simulink model "Motor_model"  (R2018a)
settings: Solver=VariableStepAuto  StartTime=0.0  StopTime=50
values from neighbouring files (symbols this model uses):
  a = Rr/Lr    (= 342.760962802)    [IM_model.m]
  b = Msr/(sigma*Ls*Lr)    (= -1.03784964259)    [IM_model.m]
  c = f/J    (= 0.00909090909091)    [IM_model.m]
  gamma = ((Lr^2)*Rs+Msr^2)/(sigma*Ls*(Lr^2))    (= -33.4582958771)    [IM_model.m]
  J = 0.011    [IM_model.m]    (also in transfer_function.m)
  m = p*Msr/(J*Lr)    (= 2899.38130148)    [IM_model.m]
  m1 = 1/(sigma*Ls)    (= -0.0325414140802)    [IM_model.m]
  Msr = 0.9644789    [IM_model.m]    (also in transfer_function.m)
  p = 1    [IM_model.m]    (also in transfer_function.m)
  ws = 2*pi*fs    (= 314.159265359)    [IM_model.m]
libraries: powerlib_meascontrol x3, powerlib x1
settings Model: Creator=ali  LastModifiedBy=ali

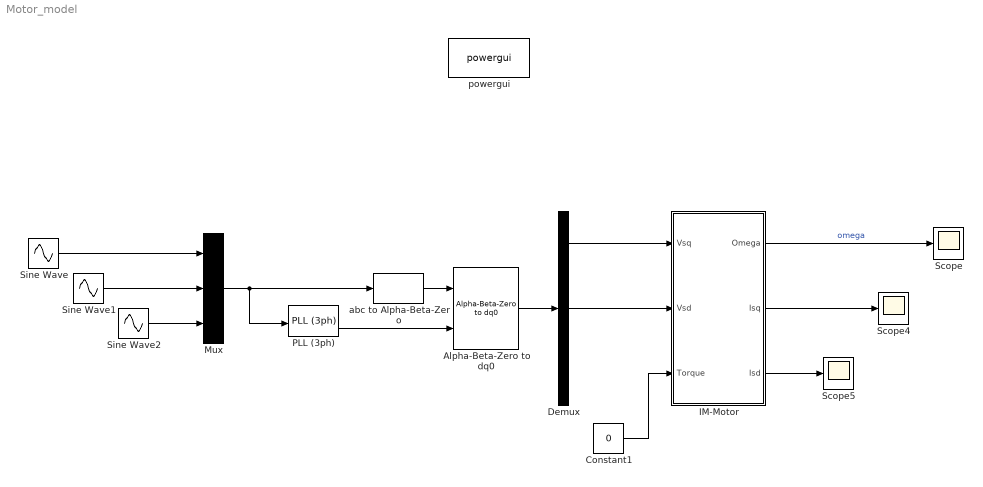
== system Motor_model ==
  Alpha-Beta-Zero to dq0 : powerlib_meascontrol/Transformations/Alpha-Beta-Zero to dq0  Alignment=90 degrees behind phase A axis
      settings: SourceProductName=Simscape Power Systems
  Constant1 : Constant  Value=0
  Demux : Demux  Outputs=3
  IM-Motor : Subsystem
  Mux : Mux  Inputs=3
  PLL (3ph) : powerlib_meascontrol/PLL/PLL (3ph)  Fmin=45  Par_Init=[0, 50]  ParK=[180, 3200, 1]  TcD=1e-4  MaxRateChangeFreq=12  FilterCutOffFreq=25  Ts=0  AGC=on
  Scope : Scope
  Scope4 : Scope
  Scope5 : Scope
  Sine Wave : Sin  Amplitude=220*sqrt(2)  Frequency=2*pi*50  SampleTime=0
  Sine Wave1 : Sin  Amplitude=220*sqrt(2)  Frequency=2*pi*50  Phase=(-120)*(2*pi/360)  SampleTime=0
  Sine Wave2 : Sin  Amplitude=220*sqrt(2)  Frequency=2*pi*50  Phase=(-240)*(2*pi/360)  SampleTime=0
  abc to Alpha-Beta-Zero : powerlib_meascontrol/Transformations/abc to Alpha-Beta-Zero
      settings: SourceProductName=Simscape Power Systems
  powergui : powerlib/powergui  Priority=1  SimulationMode=Continuous  SampleTime=50e-6  frequency=60  Iterations=50  frequencyindice=60  Pbase=100e6  ErrMax=1e-4  UnitsV=kV  UnitsW=MW  buscounter=0  FunctionMessages=off  echomessages=off  EnableUseOfTLC=off  CurrentSourceSwitches=off  DisableSnubberDevices=off  DisableRonSwitches=off  DisableVfSwitches=off  DisplayEquations=off  SolverType=Tustin/Backward Euler (TBE)  Interpol=off  ExternalGateDelay=off  methode=off  Ts=100  x0status=blocks  SPID=on  SwTol=0  HookPort=off  RestoreLinks=warning  ResistiveCurrentMeasurement=off  Frange=[0:2:500]  Ylog=off  Xlog=on  ShowGrid=off  save=off  variable=ZData  structure=0  ZoomFFT=off  StartTime=0.0  cycles=1  DisplayStyle=1  fundamental=60  FreqAxis=off  MaxFrequency=1000  frequencyindicesteady=1  RmsSteady=1  display=off
  wires:
  IM-Motor/1(Omega) -> Scope/1  "omega"
  Sine Wave/1 -> Mux/1
  Sine Wave1/1 -> Mux/2
  Sine Wave2/1 -> Mux/3
  Constant1/1 -> IM-Motor/3(Torque)
  Mux/1 -> abc to Alpha-Beta-Zero/1, PLL (3ph)/1
  abc to Alpha-Beta-Zero/1 -> Alpha-Beta-Zero to dq0/1
  PLL (3ph)/2 -> Alpha-Beta-Zero to dq0/2
  IM-Motor/2(Isq) -> Scope4/1
  IM-Motor/3(Isd) -> Scope5/1
  Alpha-Beta-Zero to dq0/1 -> Demux/1
  Demux/1 -> IM-Motor/1(Vsq)
  Demux/2 -> IM-Motor/2(Vsd)

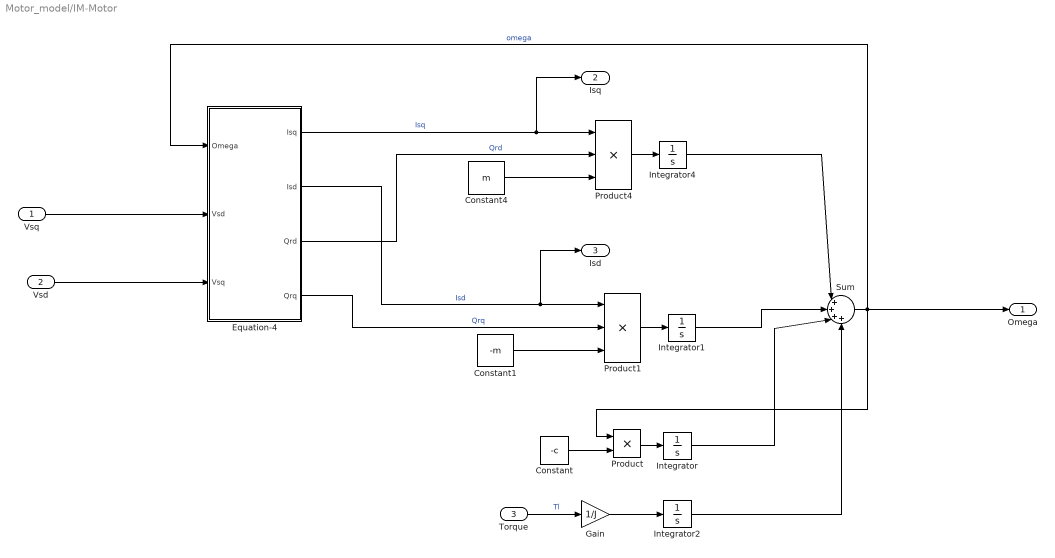
== system Motor_model/IM-Motor ==
  Vsq : Inport
  Vsd : Inport  Port=2
  Torque : Inport  Port=3
  Constant : Constant  Value=-c
  Constant1 : Constant  Value=-m
  Constant4 : Constant  Value=m
  Equation-4 : Subsystem
  Gain : Gain  Gain=1/J
  Integrator{,1..2,4} (4 alike) : Integrator
  Product : Product
  Product1 : Product  Inputs=3
  Product4 : Product  Inputs=3
  Sum : Sum  Inputs=|++++
  Omega : Outport
  Isq : Outport  Port=2
  Isd : Outport  Port=3
  wires:
  Equation-4/1(Isq) -> Isq/1, Product4/1  "Isq"
  Product/1 -> Integrator/1
  Sum/1 -> Omega/1, Equation-4/1(Omega), Product/1  "omega"
  Integrator/1 -> Sum/3
  Integrator4/1 -> Sum/1
  Constant/1 -> Product/2
  Integrator1/1 -> Sum/2
  Equation-4/3(Qrd) -> Product4/2  "Qrd"
  Vsq/1 -> Equation-4/2(Vsd)
  Equation-4/2(Isd) -> Isd/1, Product1/1  "Isd"
  Vsd/1 -> Equation-4/3(Vsq)
  Constant4/1 -> Product4/3
  Equation-4/4(Qrq) -> Product1/2  "Qrq"
  Product4/1 -> Integrator4/1
  Constant1/1 -> Product1/3
  Product1/1 -> Integrator1/1
  Integrator2/1 -> Sum/4
  Gain/1 -> Integrator2/1
  Torque/1 -> Gain/1  "Tl"

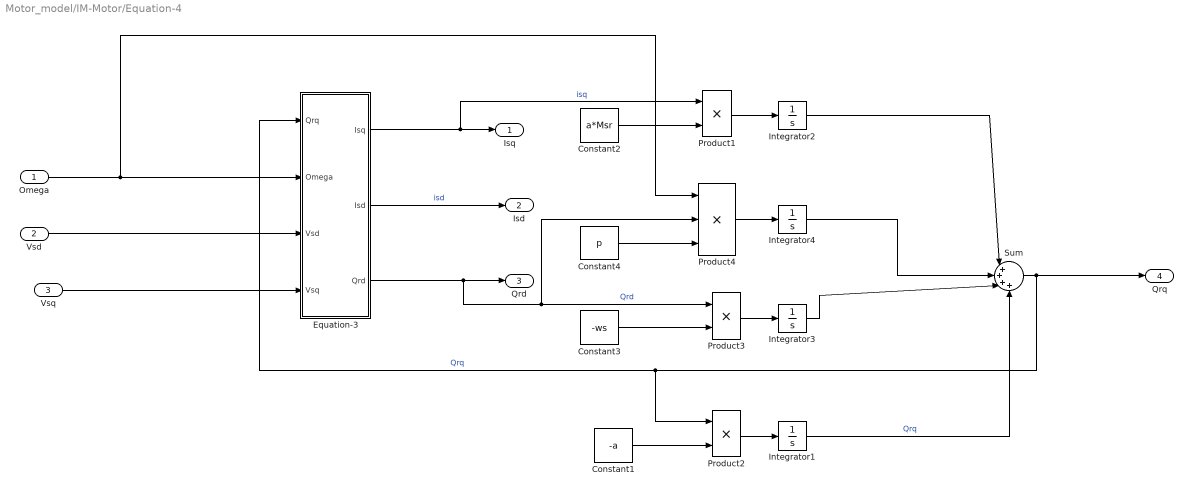
== system Motor_model/IM-Motor/Equation-4 ==
  Omega : Inport
  Vsd : Inport  Port=2
  Vsq : Inport  Port=3
  Constant1 : Constant  Value=-a
  Constant2 : Constant  Value=a*Msr
  Constant3 : Constant  Value=-ws
  Constant4 : Constant  Value=p
  Equation-3 : Subsystem
  Integrator{1..4} (4 alike) : Integrator
  Product1 : Product
  Product2 : Product
  Product3 : Product
  Product4 : Product  Inputs=3
  Sum : Sum  Inputs=|++++
  Isq : Outport
  Isd : Outport  Port=2
  Qrd : Outport  Port=3
  Qrq : Outport  Port=4
  wires:
  Product3/1 -> Integrator3/1
  Equation-3/3(Qrd) -> Qrd/1, Product4/2, Product3/1  "Qrd"
  Product2/1 -> Integrator1/1
  Constant2/1 -> Product1/2
  Sum/1 -> Qrq/1, Product2/1, Equation-3/1(Qrq)  "Qrq"
  Integrator2/1 -> Sum/1
  Omega/1 -> Product4/1, Equation-3/2(Omega)
  Integrator4/1 -> Sum/2
  Constant3/1 -> Product3/2
  Integrator3/1 -> Sum/3
  Product1/1 -> Integrator2/1
  Integrator1/1 -> Sum/4  "Qrq"
  Constant4/1 -> Product4/3
  Vsd/1 -> Equation-3/3(Vsd)
  Vsq/1 -> Equation-3/4(Vsq)
  Equation-3/2(Isd) -> Isd/1  "isd"
  Equation-3/1(Isq) -> Isq/1, Product1/1  "isq"
  Product4/1 -> Integrator4/1
  Constant1/1 -> Product2/2

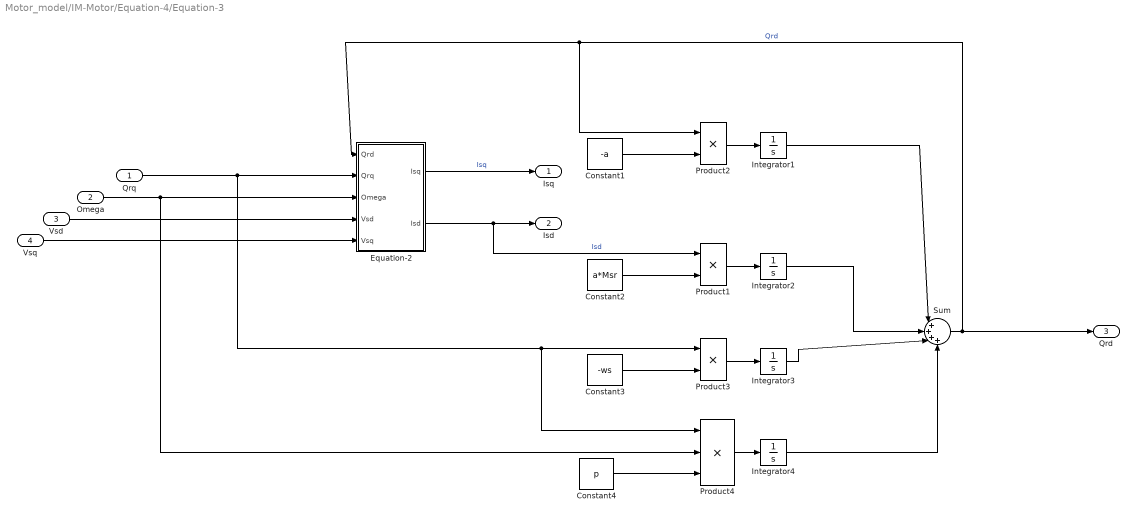
== system Motor_model/IM-Motor/Equation-4/Equation-3 ==
  Qrq : Inport
  Omega : Inport  Port=2
  Vsd : Inport  Port=3
  Vsq : Inport  Port=4
  Constant1 : Constant  Value=-a
  Constant2 : Constant  Value=a*Msr
  Constant3 : Constant  Value=-ws
  Constant4 : Constant  Value=p
  Equation-2 : Subsystem
  Integrator{1..4} (4 alike) : Integrator
  Product1 : Product
  Product2 : Product
  Product3 : Product
  Product4 : Product  Inputs=3
  Sum : Sum  Inputs=|++++
  Isq : Outport
  Isd : Outport  Port=2
  Qrd : Outport  Port=3
  wires:
  Vsd/1 -> Equation-2/4(Vsd)
  Product4/1 -> Integrator4/1
  Qrq/1 -> Equation-2/2(Qrq), Product4/1, Product3/1
  Sum/1 -> Qrd/1, Equation-2/1(Qrd), Product2/1  "Qrd"
  Integrator2/1 -> Sum/2
  Integrator1/1 -> Sum/1
  Omega/1 -> Product4/2, Equation-2/3(Omega)
  Integrator3/1 -> Sum/3
  Equation-2/2(Isd) -> Isd/1, Product1/1  "Isd"
  Integrator4/1 -> Sum/4
  Constant2/1 -> Product1/2
  Constant4/1 -> Product4/3
  Product3/1 -> Integrator3/1
  Constant3/1 -> Product3/2
  Constant1/1 -> Product2/2
  Equation-2/1(Isq) -> Isq/1  "Isq"
  Product2/1 -> Integrator1/1
  Product1/1 -> Integrator2/1
  Vsq/1 -> Equation-2/5(Vsq)

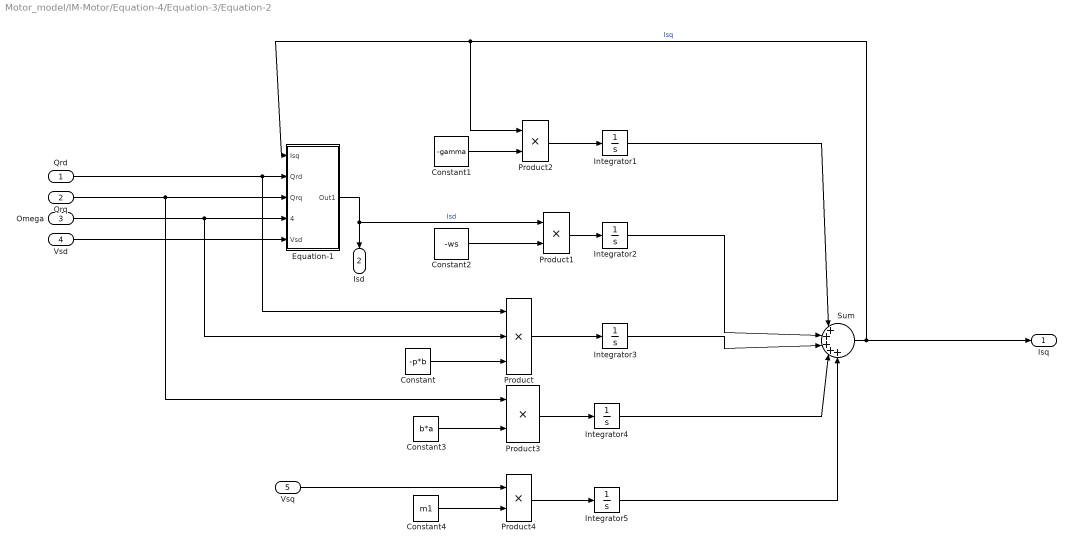
== system Motor_model/IM-Motor/Equation-4/Equation-3/Equation-2 ==
  Qrd : Inport
  Qrq : Inport  Port=2
  Omega : Inport  Port=3
  Vsd : Inport  Port=4
  Vsq : Inport  Port=5
  Constant : Constant  Value=-p*b
  Constant1 : Constant  Value=-gamma
  Constant2 : Constant  Value=-ws
  Constant3 : Constant  Value=b*a
  Constant4 : Constant  Value=m1
  Equation-1 : Subsystem
  Integrator{1..5} (5 alike) : Integrator
  Product : Product  Inputs=3
  Product{1..4} (4 alike) : Product
  Sum : Sum  Inputs=|+++++
  Isq : Outport
  Isd : Outport  Port=2
  wires:
  Qrd/1 -> Product/1, Equation-1/2(Qrd)
  Constant3/1 -> Product3/2
  Sum/1 -> Isq/1, Product2/1, Equation-1/1(Isq)  "Isq"
  Integrator5/1 -> Sum/5
  Product1/1 -> Integrator2/1
  Omega/1 -> Product/2, Equation-1/4(Omega)
  Equation-1/1(Out1) -> Isd/1, Product1/1  "Isd"
  Qrq/1 -> Product3/1, Equation-1/3(Qrq)
  Vsd/1 -> Equation-1/5(Vsd)
  Constant4/1 -> Product4/2
  Integrator3/1 -> Sum/3
  Constant2/1 -> Product1/2
  Integrator4/1 -> Sum/4
  Product4/1 -> Integrator5/1
  Product3/1 -> Integrator4/1
  Vsq/1 -> Product4/1
  Constant/1 -> Product/3
  Product/1 -> Integrator3/1
  Constant1/1 -> Product2/2
  Product2/1 -> Integrator1/1
  Integrator2/1 -> Sum/2
  Integrator1/1 -> Sum/1

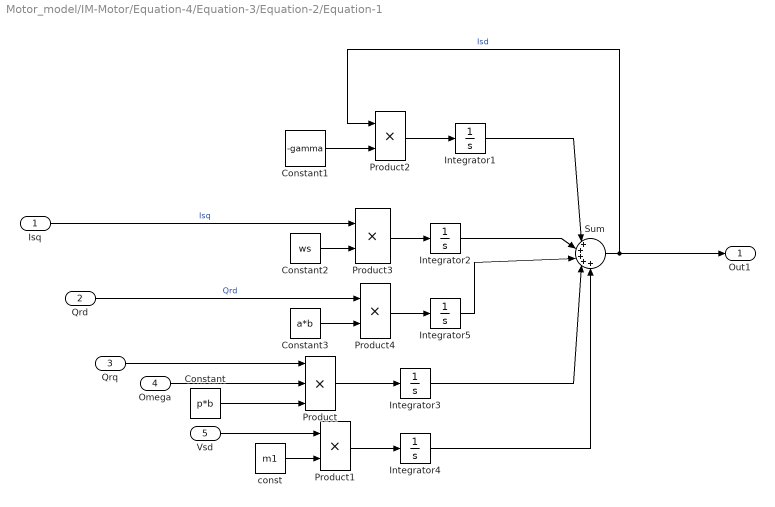
== system Motor_model/IM-Motor/Equation-4/Equation-3/Equation-2/Equation-1 ==
  Isq : Inport
  Qrd : Inport  Port=2
  Qrq : Inport  Port=3
  Omega : Inport  Port=4
  Vsd : Inport  Port=5
  Constant : Constant  Value=p*b
  Constant1 : Constant  Value=-gamma
  Constant2 : Constant  Value=ws
  Constant3 : Constant  Value=a*b
  Integrator{1..5} (5 alike) : Integrator
  Product : Product  Inputs=3
  Product{1..4} (4 alike) : Product
  Sum : Sum  Inputs=|+++++
  const : Constant  Value=m1
  Out1 : Outport
  wires:
  Product1/1 -> Integrator4/1
  Product/1 -> Integrator3/1
  Constant2/1 -> Product3/2
  Constant1/1 -> Product2/2
  Vsd/1 -> Product1/1
  Integrator1/1 -> Sum/1
  const/1 -> Product1/2
  Product4/1 -> Integrator5/1
  Integrator2/1 -> Sum/2
  Qrd/1 -> Product4/1  "Qrd"
  Constant3/1 -> Product4/2
  Integrator3/1 -> Sum/4
  Integrator5/1 -> Sum/3
  Isq/1 -> Product3/1  "Isq"
  Constant/1 -> Product/3
  Sum/1 -> Out1/1, Product2/1  "Isd"
  Product2/1 -> Integrator1/1
  Omega/1 -> Product/2
  Product3/1 -> Integrator2/1
  Integrator4/1 -> Sum/5
  Qrq/1 -> Product/1
